simulink model "sf_boiler"  (Simulink 6.0)
settings: Solver=ode45  StartTime=0.0  StopTime=1400  RelTol=1e-3
libraries: fixpt_lib_4 x1, simulink x1
settings Model: CovMetricSettings=dcmtr  Creator=The MathWorks Inc.  LastModifiedBy=batserve  ExtModeTrigMode=oneshot  ExtModeArmWhenConnect=off  ExtModeAutoUpdateStatusClock=off  ProdHWDeviceType=ASIC/FPGA
settings DataIOCC: LimitDataPoints=off  SaveOutput=off  SaveTime=off  SignalLoggingName=sigsOut
settings OptimizationCC: BlockReduction=off  BooleanDataType=off  InlineInvariantSignals=off  OptimizeModelRefInitCode=on  LifeSpan=1
settings DebuggingCC: CheckExecutionContextPreStartOutputMsg=on  CheckExecutionContextRuntimeOutputMsg=on  SolverPrmCheckMsg=none
settings HardwareCC: ProdHWDeviceType=ASIC/FPGA  TargetUnknown=on
settings RTWCC: SystemTargetFile=ert.tlc  GenCodeOnly=on  TemplateMakefile=ert_default_tmf  GenerateReport=on  RTWVerbose=off  ProcessScript=ert_make_rtw_hook  IncludeHyperlinkInReport=on  LaunchReport=on
settings CodeAppCC: IgnoreCustomStorageClasses=off
settings ERTTargetCC: TargetFcnLib=ansi_tfl_tmw.mat  GenFloatMathFcnCalls=ANSI_C  GenerateSampleERTMain=on  SupportContinuousTime=on  SupportNonInlinedSFcns=on  InlinedParameterPlacement=NonHierarchical  RootIOFormat=Individual Arguments  ERTCustomFileTemplate=example_file_process.tlc  InitialValueSource=Model

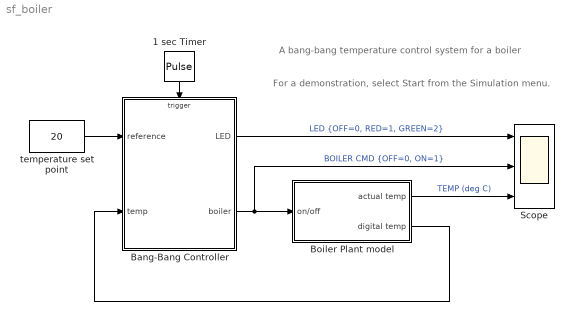
== system sf_boiler ==
  note: A bang-bang temperature control
      | system for a boiler
  note: For a demonstration, select Start from the Simulation menu.
  1 sec Timer : DiscretePulseGenerator  Orientation=down  Amplitude=int8(1)
  Bang-Bang Controller : Stateflow chart  TreatAsAtomicUnit=on  PropExecContextAcrossSSBoundary=on
  Boiler Plant model : Subsystem  PropExecContextAcrossSSBoundary=on
  Scope : Scope  NumInputPorts=3
      settings: YMin=0~0~15  YMax=2~1~24
  temperature set point : Constant  Value=20
  wires:
  1 sec Timer/1 -> Bang-Bang Controller/Trigger
  Bang-Bang Controller/2(boiler) -> Scope/2, Boiler Plant model/1(on/off)  "BOILER CMD {OFF=0, ON=1}"
  temperature set point/1 -> Bang-Bang Controller/1(reference)
  Boiler Plant model/2(digital temp) -> Bang-Bang Controller/2(temp)
  Boiler Plant model/1(actual temp) -> Scope/3  "TEMP (deg C)"
  Bang-Bang Controller/1(LED) -> Scope/1  "LED {OFF=0, RED=1, GREEN=2}"

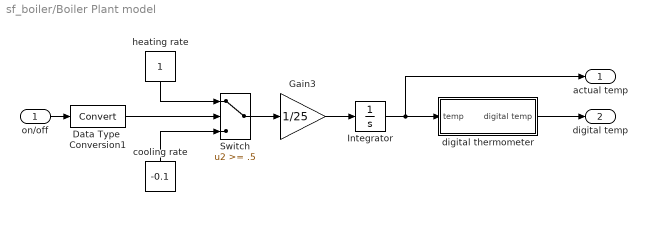
== system sf_boiler/Boiler Plant model ==
  on/off : Inport  Port=1  LatchInput=off
  Data Type  Conversion1 : DataTypeConversion  OutDataTypeMode=boolean  SaturateOnIntegerOverflow=on  RndMeth=Zero
  Gain3 : Gain  Gain=1/25  SaturateOnIntegerOverflow=on
  Integrator : Integrator  InitialCondition=15  ZeroCross=off
  Switch : Switch  Threshold=.5  SaturateOnIntegerOverflow=on  InputSameDT=on
  cooling rate : Constant  Orientation=up  Value=-0.1
  digital thermometer : Subsystem  PropExecContextAcrossSSBoundary=on
  heating rate : Constant  Orientation=down
  actual temp : Outport
  digital temp : Outport  Port=2
  wires:
  Gain3/1 -> Integrator/1
  cooling rate/1 -> Switch/3
  heating rate/1 -> Switch/1
  Switch/1 -> Gain3/1
  on/off/1 -> Data Type  Conversion1/1
  Data Type  Conversion1/1 -> Switch/2
  Integrator/1 -> actual temp/1, digital thermometer/1(temp)
  digital thermometer/1(digital temp) -> digital temp/1

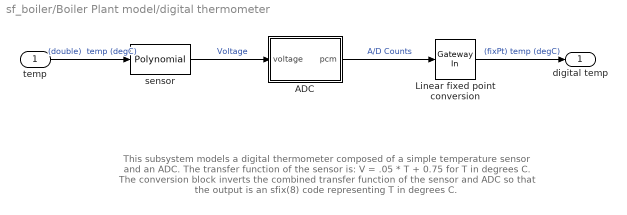
== system sf_boiler/Boiler Plant model/digital thermometer ==
  note: This subsystem models a digital thermometer composed of a simple
      | temperature sensor and an ADC.  The transfer function of the sensor is:
      | V = .05 * T + 0.75
      | for T in degrees C.
      |
      | The conversion block inverts the combined transfer function of the sensor
      | and ADC so that the output is an sfix(8) code representing T in degrees C.
  temp : Inport  Port=1  LatchInput=off
  ADC : Subsystem  PropExecContextAcrossSSBoundary=on
      mask Display: fprintf('ADC\n8-bit\n0-5V');
  Linear fixed point conversion : fixpt_lib_4/Data Type/Gateway In  InRealWorld=Stored Integer  OutputDataTypeScalingMode=Specify via dialog  OutDataType=sfix(8)  OutScaling="[ 5/256/0.05     -0.75/0.05 ]"  DoSatur=off
  sensor : simulink/Math Operations/Polynomial  coefs="[ 0.05     0.75 ]"
  digital temp : Outport
  wires:
  sensor/1 -> ADC/1(voltage)  "Voltage"
  ADC/1(pcm) -> Linear fixed point conversion/1  "A/D Counts"
  temp/1 -> sensor/1  "(double)  temp (degC)"
  Linear fixed point conversion/1 -> digital temp/1  "(fixPt) temp (degC)"

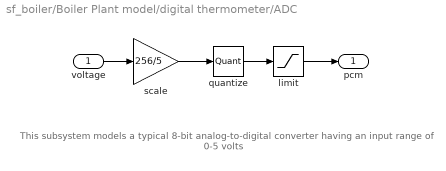
== system sf_boiler/Boiler Plant model/digital thermometer/ADC ==
  note: This subsystem models a typical
      | 8-bit analog-to-digital converter
      | having an input range of 0-5 volts
  voltage : Inport  Port=1  LatchInput=off
  limit : Saturate  UpperLimit=255  LowerLimit=0
  quantize : Quantizer  QuantizationInterval=1
  scale : Gain  Gain=256/5  SaturateOnIntegerOverflow=on
  pcm : Outport
  wires:
  limit/1 -> pcm/1
  scale/1 -> quantize/1
  quantize/1 -> limit/1
  voltage/1 -> scale/1

== stateflow chart Bang-Bang Controller ==
  state Heater [group]
    state Off
      entry: turn_boiler(OFF)
      on every(5,sec): flash_LED()
    state On
      en: turn_boiler(ON)
      du: flash_LED()
      (history)
      state HIGH
      state NORM
      state b = warm() [function]
        (default) -> (junction 22) : {b = !cold()}
      (default) -> HIGH
      HIGH -> NORM : [warm()]
    (default) -> Off
    On -> Off : after(20,sec)
    Off -> On : after(40,sec)
        | [cold()]
    NORM -> Off : [Heater.On.warm()]
  state flash_LED() [function]
    (junction 18) -> (junction 12) : {LED=OFF}
    (default) -> (junction 18)
    (junction 18) -> (junction 19) : [LED==OFF]
    (junction 19) -> (junction 23) : {LED=color}
  state turn_boiler(mode) [function]
    (default) -> (junction 13)
    (junction 13) -> (junction 14) : [mode==ON]
    (junction 16) -> (junction 15)
    (junction 14) -> (junction 16) : {color=GREEN}
    (junction 13) -> (junction 24) : {color=RED}
    (junction 15) -> (junction 17) : {LED=color;
        |  boiler=mode}
    (junction 24) -> (junction 15)
  state b = cold() [function]
    (default) -> (junction 20) : { b = temp<=reference}
  data: mode function_input int8; b function_output boolean; b function_output boolean; LED output int8; boiler output int8; color local int8; reference input fixpt; GREEN constant int8 =2; OFF constant int8; ON constant int8 =1; RED constant int8 =1; temp input fixpt
  events: sec input RISING_EDGE_EVENT
